simulink library "fuzwiz"  (Simulink 4.00)
settings Model: Creator=pascal  LastModifiedBy=pascal

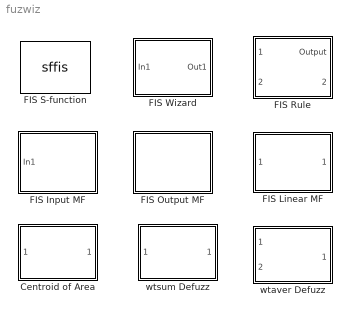
== system fuzwiz ==
  Centroid of Area : Subsystem  mask(COA Defuzzification){range=}
      mask prompts: range "Output Range:"
      mask init:
      | Xdata = linspace(range(1),range(2),101);
      settings: RTWFcnNameOpts=Auto  RTWFileNameOpts=Auto
      mask Display: disp('COA')
  FIS Input MF : Subsystem  mask(Input MF Eval){fis=, j_in=}
      mask prompts: fis "FIS structure:"; j_in "Input:"
      mask init:
      | fuzwizmask(gcb,fis,j_in)
      settings: RTWFcnNameOpts=Auto  RTWFileNameOpts=Auto
      mask Display: disp('Input MF')
  FIS Linear MF : Subsystem  mask(Linear Output MF){a=, b=}
      mask prompts: a "Linear Coefficients:"; b "Constant Coefficients:"
      settings: RTWFcnNameOpts=Auto  RTWFileNameOpts=Auto
      mask Display: disp('Linear MF')
  FIS Output MF : Subsystem  mask(Output MF Eval){fis=, j_out=}
      mask prompts: fis "FIS structure:"; j_out "Output:"
      mask init:
      | fuzwizmask(gcb,fis,j_out)
      settings: RTWFcnNameOpts=Auto  RTWFileNameOpts=Auto
      mask Display: disp('Output MF')
  FIS Rule : Subsystem  mask(FIS Rule){fis=, j_rule=}
      mask prompts: fis "FIS structure:"; j_rule "Rule:"
      mask init:
      | fuzwizmask(gcb,fis,j_rule)
      settings: RTWFcnNameOpts=Auto  RTWFileNameOpts=Auto
      mask Display: disp('Rule')
  FIS S-function : S-Function  FunctionName=sffis  Parameters=fis  PortCounts=[]  SFunctionModules=sfsup
  FIS Wizard : Subsystem  mask(FIS Wizard){fis=}
      mask prompts: fis "FIS structure:"
      mask init:
      | fuzwizmask(gcb,fis);
      settings: RTWFcnNameOpts=Auto  RTWFileNameOpts=Auto
      mask Display: disp('FIS')
  wtaver Defuzz : Subsystem
      settings: RTWFcnNameOpts=Auto  RTWFileNameOpts=Auto
      mask Type: WTAVER Defuzzification
      mask Display: disp('WTAVER')
  wtsum Defuzz : Subsystem
      settings: RTWFcnNameOpts=Auto  RTWFileNameOpts=Auto
      mask Type: WTSUM Defuzzification
      mask Display: disp('WTSUM')

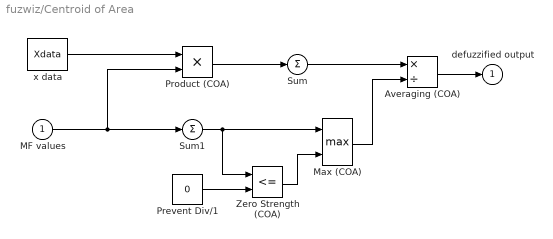
== system fuzwiz/Centroid of Area ==
  MF values : Inport  Port=1
  Averaging (COA) : Product  Inputs=*/  Multiplication=Element-wise(.*)  SaturateOnIntegerOverflow=on
  Max (COA) : MinMax  Function=max  Inputs=2
  Prevent Div/1 : Constant  Value=0
  Product (COA) : Product  Inputs=2  Multiplication=Element-wise(.*)  SaturateOnIntegerOverflow=on
  Sum : Sum  Inputs=+  SaturateOnIntegerOverflow=on
  Sum1 : Sum  Inputs=+  SaturateOnIntegerOverflow=on
  Zero Strength (COA) : RelationalOperator  Operator=<=
  x data : Constant  Value=Xdata
  defuzzified output : Outport  Port=1
  wires:
  Averaging (COA)/1 -> defuzzified output/1
  Sum/1 -> Averaging (COA)/1
  MF values/1 -> Sum1/1, Product (COA)/2
  Product (COA)/1 -> Sum/1
  x data/1 -> Product (COA)/1
  Sum1/1 -> Max (COA)/1, Zero Strength (COA)/1
  Max (COA)/1 -> Averaging (COA)/2
  Prevent Div/1/1 -> Zero Strength (COA)/2
  Zero Strength (COA)/1 -> Max (COA)/2

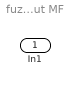
== system fuzwiz/FIS Input MF ==
  In1 : Inport  Port=1

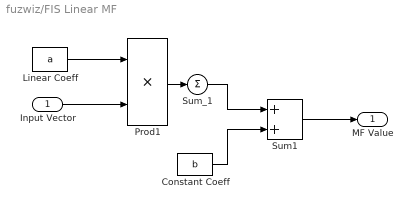
== system fuzwiz/FIS Linear MF ==
  Input Vector : Inport  Port=1
  Constant Coeff : Constant  Value=b
  Linear Coeff : Constant  Value=a
  Prod1 : Product  Inputs=2  Multiplication=Element-wise(.*)  SaturateOnIntegerOverflow=on
  Sum1 : Sum  Inputs=2  SaturateOnIntegerOverflow=on
  Sum_1 : Sum  Inputs=1  SaturateOnIntegerOverflow=on
  MF Value : Outport  Port=1
  wires:
  Linear Coeff/1 -> Prod1/1
  Prod1/1 -> Sum_1/1
  Sum_1/1 -> Sum1/1
  Constant Coeff/1 -> Sum1/2
  Input Vector/1 -> Prod1/2
  Sum1/1 -> MF Value/1

== system fuzwiz/FIS Output MF ==

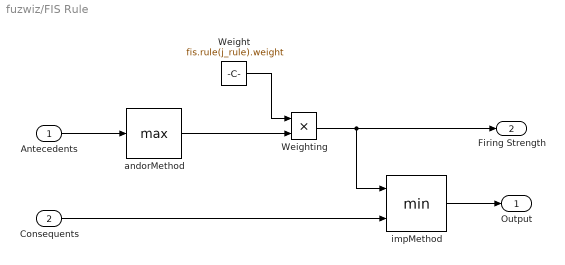
== system fuzwiz/FIS Rule ==
  Antecedents : Inport  Port=1
  Consequents : Inport  Port=2
  Weight : Constant  Value=fis.rule(j_rule).weight
  Weighting : Product  Inputs=2  Multiplication=Element-wise(.*)  SaturateOnIntegerOverflow=on
  andorMethod : MinMax  Function=max  Inputs=1
  impMethod : MinMax  Function=min  Inputs=2
  Output : Outport  Port=1
  Firing Strength : Outport  Port=2
  wires:
  Antecedents/1 -> andorMethod/1
  andorMethod/1 -> Weighting/2
  Weight/1 -> Weighting/1
  Consequents/1 -> impMethod/2
  Weighting/1 -> impMethod/1, Firing Strength/1
  impMethod/1 -> Output/1

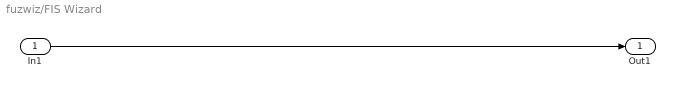
== system fuzwiz/FIS Wizard ==
  In1 : Inport  Port=1
  Out1 : Outport  Port=1
  wires:
  In1/1 -> Out1/1

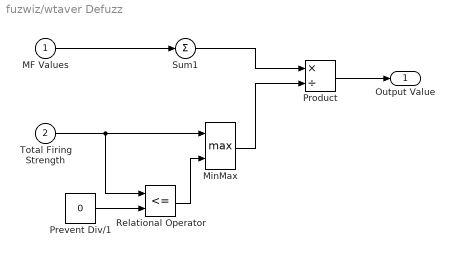
== system fuzwiz/wtaver Defuzz ==
  MF Values : Inport  Port=1
  Total Firing Strength : Inport  Port=2
  MinMax : MinMax  Function=max  Inputs=2
  Prevent Div/1 : Constant  Value=0
  Product : Product  Inputs=*/  Multiplication=Element-wise(.*)  SaturateOnIntegerOverflow=on
  Relational Operator : RelationalOperator  Operator=<=
  Sum1 : Sum  Inputs=1  SaturateOnIntegerOverflow=on
  Output Value : Outport  Port=1
  wires:
  MF Values/1 -> Sum1/1
  Sum1/1 -> Product/1
  Product/1 -> Output Value/1
  Total Firing Strength/1 -> MinMax/1, Relational Operator/1
  MinMax/1 -> Product/2
  Relational Operator/1 -> MinMax/2
  Prevent Div/1/1 -> Relational Operator/2

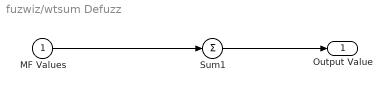
== system fuzwiz/wtsum Defuzz ==
  MF Values : Inport  Port=1
  Sum1 : Sum  Inputs=1  SaturateOnIntegerOverflow=on
  Output Value : Outport  Port=1
  wires:
  MF Values/1 -> Sum1/1
  Sum1/1 -> Output Value/1
